simulink model "TxRxRFModel"  (R2018a)
settings: Solver=VariableStepAuto  StartTime=0.0  StopTime=10.0  RelTol=1e-3
InitFcn:
  | barker = comm.BarkerCode('SamplesPerFrame', 28, 'Length', 11);
  | seq = barker()+1;
  | M = 4;
  | hPSKModTrain   = comm.PSKModulator(M, ...
  |     'PhaseOffset',pi/4, ...
  |     'SymbolMapping','Binary');
  | xPreambleSeq = hPSKModTrain(seq);
  | 
  | 
  | %%%%%%%%%%%%
  | 
  | % AGC Preamble
  | reps = 5;
  | barker = comm.BarkerCode('SamplesPerFrame', 16, 'Length', 13);
  | seq = barker()+1;
  | %preamble = zeros(16*reps,1);
  | preambleFull = repmat(seq,reps,1);
  | rctFilt = comm.RaisedCosineTransmitFilter('FilterSpanInSymbols', 128,...
  | 'RolloffFactor',0.5,...
  | 'OutputSamplesPerSymbol',4);
  | preambleFullFilt = rctFilt(preambleFull);
  | 
  | %%%%%%%%%%%%
  | 
  | %RadioSampleRate = 1e6;
  | RadioSampleRate = 20e6;
  | RadioFrameLength = 1e5;
  | 
  | VibertiTracebackLength = 34+0;
  | numTrainingSamples = 250;
  | crc32Poly = [1 0 0 0 0 0 1 0 0 1 1 0 0 0 0 0 1 0 0 0 1 1 1 0 1 1 0 1 1 0 1 1 1];
  | crcDecodeLag = length(crc32Poly)-1+2;
  | 
  | %%%%%%%%%%%%
  | 
  | beta = 0.5;
  | span = 8;
  | sps = 4;
  | filterGain = 1;
  | coeff = rcosdesign(beta, span, sps, 'sqrt')*filterGain;
  | 
  | %%%%%%%%%%%%
  | 
  | samplesPerSymbol = 4;
  | maxPacketBits = 8*1500;
  | bItsPerSymbol = 2;
  | CodeRate = 2;
  | tailSymbols = 40;
  | maxPayloadSymbols = maxPacketBits*CodeRate/bItsPerSymbol+tailSymbols;
undefined symbols (not defined in the file or in its folder): ad9361_models, ad9361_preload, ad9361_rx, ad9361_tx, D, dBval, DCLeak_Matrix, designMultirateFIR, dfilt, doppler, errordlg, Frame, fuzz_val, GainImb_Matrix, IP2_Matrix, IP3_Matrix, magnitude
libraries: simulink x24, simrfV2elements x21, simrfV2util1 x9, dsparch4 x8, simrfV2junction1 x8, dspmlti4 x7, ad9361_private x3, simrfV2sources1 x3, dspmathops x3, commchan3 x2, hdlsllib x2, commdigbbndpm3 x2
(part 1 of 3)
settings Model: SimulationMode=accelerator  Creator=tcollins  LastModifiedBy=tcollins

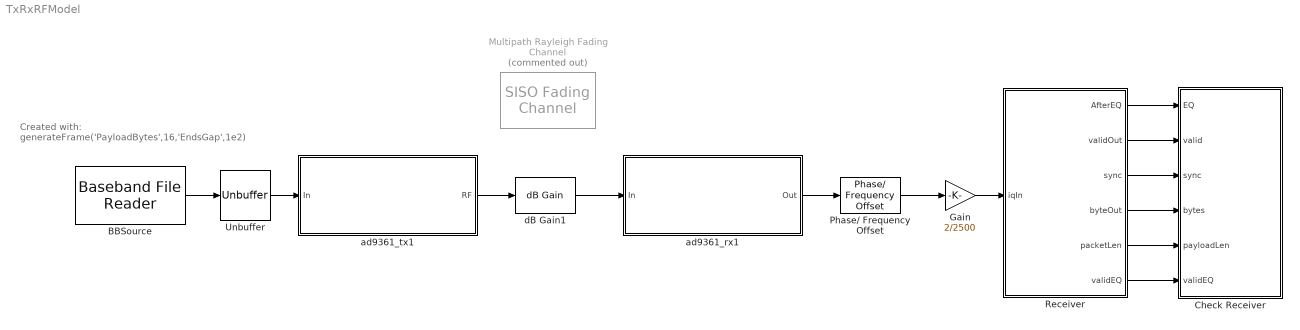
== system TxRxRFModel ==
  note: Created with:
      | generateFrame('PayloadBytes',16,'EndsGap',1e2)
  BBSource : commsource2/Baseband File Reader  Filename=refIQFrame.bb  InheritSampleTimeFromFile=off  SampleTime=100000/(RadioSampleRate)  SamplesPerFrame=100000  CyclicRepetition=on  FileEndOutputPort=off  SimulateUsing=Interpreted execution
      settings: SourceProductName=Communications Toolbox  SourceProductBaseCode=CM
  Check Receiver : Subsystem
  Gain : Gain  Gain=2/2500
  Multipath Rayleigh Fading Channel : commchan3/SISO Fading Channel  Commented=on  InheritSampleRate=on  SampleRate=1  PathDelays=[0 3e-8 5e-7]  AveragePathGains=[0 -20 -40]-60  NormalizePathGains=off  FadingDistribution=Rayleigh  KFactor=3  DirectPathDopplerShift=0  DirectPathInitialPhase=0  MaximumDopplerShift=5  DopplerSpectrum=doppler('Jakes')  ChannelInterpolationMethod=Polyphase  RandomStream=mt19937ar with seed  RandomNumGenerator=shr3cong  Seed=54873  PathGainsOutputPort=off  ChannelFilterDelayOutputPort=off  SimulateUsing=Code generation  Visualization=Off  PathsForDopplerDisplay=1  SamplesToDisplay=25%
      settings: SourceProductName=Communications Toolbox
  Phase/ Frequency Offset : commrflib2/Phase// Frequency Offset  phaseOffset=0  freqPort=off  freqOffset=1000
      settings: SourceProductName=Communications Toolbox
  Receiver : Subsystem  AncestorBlock=RxFloatingPointLibrary/Receiver
  Unbuffer : Unbuffer
  ad9361_rx1 : Subsystem  AncestorBlock=ad9361_models/ad9361_rx  LoadFcn=ad9361_preload(bdroot,'rx')  mask(ad9361_RX){TestSignal=Custom, LO=2e9, RF=2e9, Trf=1/160e6, RF_BW=160, IQ_rate=20}
      mask prompts: TestSignal "Filter Configuration:"; LO "LO Frequency [Hz]:"; RF "RF Center Frequency [Hz]:"; Trf "Step Size RF Simulation [s]:"; RF_BW "Input RF Bandwidth (MHz)"; IQ_rate "I/Q Sample Rate (MHz)"
      mask help: Model an Analog Devices ad9361 RF Receiver.
      mask init:
      | %load ad9361_rx_tables;
      | [ADIGainTable, ADIPhaseTable, ...
      |     DCLeak_Matrix, GainImb_Matrix, ...
      |     IP2_Matrix, IP3_Matrix] = ad9361_rx_gaintable(LO);
      | ad9361_rx_pars = ad9361_rx_initfcn(gcb,'Init');
      | ad9361_rx_pars = ad9361_rx_initfcn(gcb,'Build');
      mask Help:
      | Model an Analog Devices ad9361 RF Receiver. This model predicts thermal noise, spectral growth, LO carrier leakage and image signals, quantization noise in manual and slow attack control mode.
      | 
      | To change the automatic gain control mode, toggle the manual switch between manual mode and slow-attack control mode under the receiver mask. For manual mode, directly specify the index of the gain table in the constant block "manual index".
      | 
      | For signals with LTE 5MHz, LTE 10 MHz and LTE 20 MHz characteristics, the default configurations recommended by Analog Devices are directly available.
      | 
      | The filters are programmable. Use the Analog Devices Wizard App to custom design Filters. Select the option Custom in the Filter Configuration menu and click Design Filter button. The Filter Design app will open automatically. Make sure a receiver filter is designed instead of a transmitter filter. After designing the filter, click the button Export to Workspace in the App. The custom filter design is saved in the model set up. Next time a simulation is setup with custom filter configuration, the latest filter design is used.
      | 
      | Make sure that the input signal sample time and the expected step size of the RF simulation are the same. In case of a mismatch, an error is generated.
      mask TypeOptions TestSignal: 5MHz LTE | 10MHz LTE | 20MHz LTE | Custom
      mask Callback TestSignal:
      | % Set Mask visibilites and enables
      | ad9361_rx_mask_callbacks(gcb,'TestSignal')
      mask Callback Trf:
      | % block = gcb;
      | % p = Simulink.Mask.get(block);
      | % tmp = num2str(1/eval(get_param(gcb,'Trf'))/1e6,6);
      | % p.Parameters(5).Value = tmp;
      | set_param(gcb,'RF_BW',num2str(1/eval(get_param(gcb,'Trf'))/1e6,6));
      mask DialogControl ParameterGroupVar Prompt: ad9361 Receiver
      mask DialogControl Control2 Prompt: SpacerDesign
      mask DialogControl DesignFilter Prompt: Design Filter
      mask DialogControl DesignFilter Callback: ad9361_rx_initfcn(gcb,'DesignFilter');
      mask Display: text(0.5,0.5,'ad9361_RX','horizontalAlignment','center');
  ad9361_tx1 : Subsystem  AncestorBlock=ad9361_models/ad9361_tx  LoadFcn=ad9361_preload(bdroot,'tx')  mask(ad9361_TX){TestSignal=Custom, LOFreq=2e9, Att=0, IQ_rate=20, RF_BW=160}
      mask prompts: TestSignal "Filter Configuration:"; LOFreq "LO Frequency (Hz)"; Att "Attenuation (dB)"; IQ_rate "I/Q Sample Rate (MHz)"; RF_BW "RF Bandwidth (MHz)"
      mask help: Model an Analog Devices ad9361 RF Transmitter.
      mask init:
      | ad9361_tx_pars = ad9361_tx_initfcn(gcb,'Init');
      | ad9361_tx_pars = ad9361_tx_initfcn(gcb,'Build');
      mask Help:
      | Model an Analog Devices ad9361 RF Transmitter. This predicts thermal noise, phase noise, spectral growth, LO carrier leakage and image signals.
      | 
      | To change the attenuation value, modify the constant value in Attenuation block under the Transmitter mask. Transmitter attenuation is tunable between 0 to 80dB in steps of 0.25dB.
      | 
      | For signals with LTE 5MHz, LTE 10 MHz and LTE 20 MHz characteristics, the default configurations recommended by Analog Devices are directly available.
      | 
      | The filters are programmable. Use the Analog Devices Wizard App to custom design Filters. Select the option Custom in the Filter Configuration menu and click Design Filter button. The Filter Design App will open automatically. Make sure a transmitter filter is designed instead of a receiver filter. After designing the filter, click the button Export to Workspace in the App. The custom filter design is saved in the model set up. Next time a simulation is setup with custom filter configuration, the latest filter design is used.
      | 
      | Make sure that the input signal sample time and the expected signal sample time are the same. In case of a mismatch, an error is generated.
      mask TypeOptions TestSignal: 5MHz LTE | 10MHz LTE | 20MHz LTE | Custom
      mask Callback TestSignal:
      | % Control DesignFilter visibility
      | ad9361_tx_mask_callbacks(gcb,'TestSignal')
      mask DialogControl ParameterGroupVar Prompt: ad9361 Transmitter
      mask DialogControl DesignFilter Prompt: Design Filter
      mask DialogControl DesignFilter Callback: [~] = ad9361_tx_initfcn(gcb,'DesignFilter');
      mask DialogControl Control3 Prompt: SpacerDesign
      mask Display: text(0.5,0.5,'ad9361_TX','horizontalAlignment','center');
  dB Gain1 : dspmathops/dB Gain  dB=-60  intype=Amplitude
      settings: SourceProductName=DSP System Toolbox  SourceProductBaseCode=DS
  wires:
  BBSource/1 -> Unbuffer/1
  ad9361_tx1/1(RF) -> dB Gain1/1
  Unbuffer/1 -> ad9361_tx1/1(In)
  dB Gain1/1 -> ad9361_rx1/1(In)
  Phase/ Frequency Offset/1 -> Gain/1
  Receiver/1(AfterEQ) -> Check Receiver/1(EQ)
  Receiver/2(validOut) -> Check Receiver/2(valid)
  Receiver/3(sync) -> Check Receiver/3(sync)
  Receiver/4(byteOut) -> Check Receiver/4(bytes)
  Receiver/5(packetLen) -> Check Receiver/5(payloadLen)
  Receiver/6(validEQ) -> Check Receiver/6(validEQ)
  Gain/1 -> Receiver/1(iqIn)
  ad9361_rx1/1(Out) -> Phase/ Frequency Offset/1

== system TxRxRFModel/Check Receiver ==
  EQ : Inport
  valid : Inport  Port=2
  sync : Inport  Port=3
  bytes : Inport  Port=4
  payloadLen : Inport  Port=5
  validEQ : Inport  Port=6
  Constellation Diagram : Subsystem
  DMA Capture : MATLAB Function  TreatAsAtomicUnit=on
  wires:
  EQ/1 -> Constellation Diagram/1(In1)
  validEQ/1 -> Constellation Diagram/Enable
  bytes/1 -> DMA Capture/1(bytes)
  valid/1 -> DMA Capture/2(validOut)
  sync/1 -> DMA Capture/3(sync)
  payloadLen/1 -> DMA Capture/4(payloadLen)

== system TxRxRFModel/Receiver ==
  iqIn : Inport
  After SRRC : ConstellationDiagram
  CRC Check and DMA Pack : Subsystem
  Constellation Diagram : Subsystem
  Frame Recover : Subsystem
  From Radio : SpectrumAnalyzer
  Gardner Timing Recovery : Subsystem
  Raised Cosine Receive Filter : commfilt2/Raised Cosine Receive Filter  filtType=Square root  R=0.5  filtSpan=8  N=4  downFactor=1  downOffset=0  filterGain=1  RateOptions=Allow multirate processing  framing=Mute  checkCoeff=off  variableName=rcRxFilt  currentFiltSpan=8  D=(8)/2  inputOffset=0  sampMode=Mute  saveAsFlag=0  rateMode=Downsampling  checkGain=Normalized  launchFVT=on  roundingMode=Floor  overflowMode=off  coeffDataTypeStr=Inherit: Same word length as input  coeffMin=[]  coeffMax=[]  coeffLastDataTypeStr=Inherit: Same word length as input  accumDataTypeStr=Inherit: Same as product output  accumLastDataTypeStr=Inherit: Same as product output  outputDataTypeStr=Inherit: Same as accumulator  outputMin=[]  outputMax=[]  outputLastDataTypeStr=Inherit: Same as accumulator
  AfterEQ : Outport
  validOut : Outport  Port=2
  sync : Outport  Port=3
  byteOut : Outport  Port=4
  packetLen : Outport  Port=5
  validEQ : Outport  Port=6
  wires:
  Gardner Timing Recovery/1(dataOut) -> Constellation Diagram/1(In1), Frame Recover/1(dataIn)
  Gardner Timing Recovery/2(strobe) -> Constellation Diagram/Enable, Frame Recover/2(validIn), Frame Recover/Enable
  Raised Cosine Receive Filter/1 -> After SRRC/1, Gardner Timing Recovery/1(dataIn)
  iqIn/1 -> Raised Cosine Receive Filter/1
  Frame Recover/1(AfterEQ) -> AfterEQ/1
  Frame Recover/4(frameStart) -> CRC Check and DMA Pack/3(startData)
  Frame Recover/5(frameEnd) -> CRC Check and DMA Pack/4(endCRC)
  Frame Recover/3(data) -> CRC Check and DMA Pack/2(bits)
  Frame Recover/6(packetLen) -> CRC Check and DMA Pack/5(payloadLen)
  CRC Check and DMA Pack/2(validOut) -> validOut/1
  CRC Check and DMA Pack/1(byteOut) -> byteOut/1
  CRC Check and DMA Pack/3(sync) -> sync/1
  CRC Check and DMA Pack/4(payloadLenOut) -> packetLen/1
  Frame Recover/2(validOut) -> validEQ/1, CRC Check and DMA Pack/1(validIn)

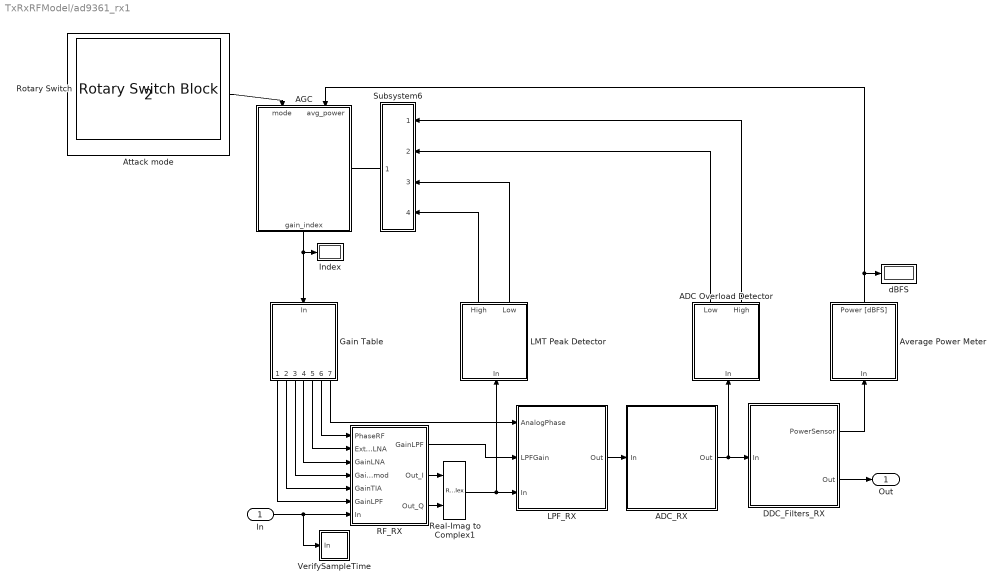
== system TxRxRFModel/ad9361_rx1 ==
  In : Inport
  ADC Overload Detector : Subsystem  mask{Ncycles=4, Lthreshold=47, Hthreshold=58}
      mask prompts: Ncycles "Number of Integration Cycles"; Lthreshold "Low Threshold"; Hthreshold "High Threshold"
      mask DialogControl DescGroupVar Prompt: ADC Overload Detector
  ADC_RX : Subsystem
  AGC : Stateflow chart  TreatAsAtomicUnit=on  mask{T=1, PeakOverLoadWait=1, SettlingDelay=32, FIR_Ts=ad9361_rx_pars.Tadc*ad9361_rx_pars.HB_interp, LMT_G_dec_fast=2, ADC_G_dec_fast=2, AGC_G_dec_fast=1, AGC_G_dec_slow=1, AGC_G_inc_fast=1, AGC_G_inc_slow=1, ManualGainIndex=76, C=3072 %approx 0.2ms, N_LMT_H=10, N_LMT_L=10, N_ADC_H=10, N_ADC_L=10, PT_HH=-8, PT_H=-10, PT_L=-12, PT_LL=-15, AGC_lock_level=-10, Max_Increase=5, EnableIncrGain=1, EnableGainIncAfterLock=1, AGC_attack_delay=10, EnergyDetectCount=32, IncrTime=5, LowPower=-13, PostLockStepSize=1, PowerMeasDuration=64, GainReset=Max Gain, GainOffset=5, EnergyLost=1, StrongerSignalThreshold=10, GainLockExitCount=8, Overrange=8}
      mask prompts: T "Extra delay margin [us]"; PeakOverLoadWait "Peak Overload Wait Time [cycles]"; SettlingDelay "Settling Delay Power Meter [cycles]"; FIR_Ts "FIR Input Clock Time"; LMT_G_dec_fast "LMT peak large decrement"; ADC_G_dec_fast "ADC peak large decrement"; AGC_G_dec_fast "Average Power large decrement"; AGC_G_dec_slow "Average Power small decrement"; AGC_G_inc_fast "Average Power large increment"; AGC_G_inc_slow "Average Power small increment"; ManualGainIndex "Gain Index"; C "Gain Update Counter [cycles]"; N_LMT_H "LMT Upper Count"; N_LMT_L "LMT Lower Count"; N_ADC_H "ADC Upper Count"; N_ADC_L "ADC Lower Count"; PT_HH "Outer Threshold High [dBFS]"; PT_H "Inner Threshold High [dBFS]"; PT_L "Inner Threshold Low [dBFS]"; PT_LL "Outer Threshold Low [dBFS]"; AGC_lock_level "AGC Lock Level [dBFS]"; Max_Increase "AGC Lock Level Max Increase [Index]"; EnableIncrGain "Enable Gain Increment [0/1]"; EnableGainIncAfterLock "Enable Gain Increment After Gain Lock [0/1]"; AGC_attack_delay "Attack delay [us]"; EnergyDetectCount "Energy Detect Count [cycles]"; IncrTime "Increment Time [cycles]"; LowPower "Low Power Threshold"; PostLockStepSize "Post Lock Level Step Size [Index]"; PowerMeasDuration "Power Measurement Duration - State 5 [cycles]"; GainReset "Gain Index When Reset"; GainOffset "Optimize Gain Offset"; EnergyLost "Energy Lost Level [dB]"; StrongerSignalThreshold "Stronger Signal Threshold [dB]"; GainLockExitCount "Gain Lock Exit Count [cycles]"; Overrange "Overrange Count [Events]"
      mask init:
      | EnergyDetectCount = EnergyDetectCount*FIR_Ts;
      | C = C*FIR_Ts;
      | SettlingDelay = SettlingDelay*FIR_Ts;
      | PeakOverLoadWait = PeakOverLoadWait*FIR_Ts;
      | PowerMeasDuration = PowerMeasDuration*FIR_Ts;
      | IncrTime = IncrTime*FIR_Ts;
      | 
      | tmp = get_param(gcb,'parent');
      | n = get_param([tmp, '/Average Power Meter'], 'Ncycles');
      | DecPowerMeasDuration = str2num(n)*FIR_Ts;
  Attack mode : Constant  Value=2  SampleTime=-1
      mask Display: disp(' ')
  Average Power Meter : Subsystem  mask{Ncycles=64}
      mask prompts: Ncycles "Number of Integration Cycles"
      mask DialogControl DescGroupVar Prompt: Average Power Meter
  DDC_Filters_RX : Subsystem
  Gain Table : Subsystem
  "Index " : Display
  LMT Peak Detector : Subsystem  mask{HThreshold=800, LThreshold=704}
      mask prompts: HThreshold "High Threshold [mV]"; LThreshold "Low Threshold [mV]"
      mask DialogControl DescGroupVar Prompt: LMT Peak Detector
  LPF_RX : Subsystem
  RF_RX : Subsystem  mask{RF=RF, LO=LO, Tstep=Trf}
      mask prompts: RF "Center Frequency [Hz]"; LO "LO Frequency [Hz]"; Tstep "Sample Time [s]"
      mask init:
      | freq = [0.8e9, 2.4e9, 5.5e9];
      | nf   = [2,     3,     3.8];
      | NF   = interp1(freq, nf, LO,'linear','extrap');
      | 
      | if length(unique([RF LO])) == 2
      |     HB = [3 1];
      | else
      |     HB = 3;
      | end
      mask DialogControl DescGroupVar Prompt: ad9361 Receiver RF Front End
  Real-Imag to Complex1 : RealImagToComplex
  Rotary Switch : RotarySwitchBlock  WebBlockId=5998  LabelPosition=Hide
      settings: Values={{'Slow', 'Manual', 'Fast'}, [0 1 2]}
  Subsystem6 : Subsystem  mask{NCyclesADC=4}
      mask prompts: NCyclesADC "ADC Integration Cycles"
  VerifySampleTime : Subsystem
  dBFS : Display
  Out : Outport
  wires:
  Gain Table/6(RF phase) -> RF_RX/1(PhaseRF)
  RF_RX/2(Out_I) -> Real-Imag to Complex1/1
  RF_RX/3(Out_Q) -> Real-Imag to Complex1/2
  Real-Imag to Complex1/1 -> LMT Peak Detector/1(In), LPF_RX/3(In)
  Gain Table/2(tia) -> RF_RX/5(GainTIA)
  Gain Table/3(demod) -> RF_RX/4(GainDemod)
  Gain Table/4(lna) -> RF_RX/3(GainLNA)
  LPF_RX/1(Out) -> ADC_RX/1(In)
  LMT Peak Detector/2(Low) -> Subsystem6/3(LMT_L)
  Gain Table/1(lpf) -> RF_RX/6(GainLPF)
  DDC_Filters_RX/1(PowerSensor) -> Average Power Meter/1(In)
  ADC Overload Detector/2(High) -> Subsystem6/1(ADC_H)
  LMT Peak Detector/1(High) -> Subsystem6/4(LMT_H)
  ADC Overload Detector/1(Low) -> Subsystem6/2(ADC_L)
  DDC_Filters_RX/2(Out) -> Out/1
  In/1 -> RF_RX/7(In), VerifySampleTime/1(In)
  Subsystem6/1(Peak) -> AGC/Trigger
  RF_RX/1("GainLPF ") -> LPF_RX/2(LPFGain)
  Gain Table/5(External LNA) -> RF_RX/2(ExternalLNA)
  Attack mode/1 -> AGC/1(mode)
  Average Power Meter/1(Power [dBFS]) -> dBFS/1, AGC/2(avg_power)
  AGC/1(gain_index) -> "Index "/1, Gain Table/1(In)
  ADC_RX/1(Out) -> DDC_Filters_RX/1(In), ADC Overload Detector/1(In)
  Gain Table/7(Analog phase) -> LPF_RX/1(AnalogPhase)

== system TxRxRFModel/ad9361_tx1 ==
  In : Inport
  Analog_Filters_TX : Subsystem
  Attenuation : Constant  Value=Att
  DUC_Filters_TX : Subsystem
  RF_TX : Subsystem  mask{RF=LOFreq, Tstep=ad9361_tx_pars.Tduc}
      mask prompts: RF "Center Frequency (Hz)"; Tstep "Sample Time (s)"
      mask init:
      | Gain = interp1([800e6, 2.4e9, 5.5e9], [0, 0, -1]+8.3, RF, 'linear', 'extrap');
      | 
      | % Output referred IP3
      | oip3_800MHz = [23, 25, 10, 10];
      | oip3_2p4GHz = [19, 18,  6,  6];
      | oip3_5p5GHz = [17, 13,  2,  2];
      | Att_ip3     = [0 4 20 80];
      | if RF < 1.6e9
      |     OIP3v = oip3_800MHz;
      | elseif RF < 4e9
      |     OIP3v = oip3_2p4GHz;
      | else
      |     OIP3v = oip3_5p5GHz;
      | end
      | % Attenuation measurement data (dB)
      | Attdata  = [0  10  20  30  40  50   60   70   80];
      | % LO carrier leakage (dBm)
      | LO_leak  = ([-58 -52 -60 -71 -81 -82 -101 -102 -100]-Gain-6)/10;
      | % Gain imbalance (dBc)
      | Gain_imb = [-55.5 -66.2 -53.5 -57.5 -44.5 -46.3 -54.2 -46.1 -34.3]/20;
      | % Phase noise characteristics (dBm/Hz)
      | freqPN   = [1e3, 1e4, 1e5, 1e6, 3e6];
      | PN       = [-95, -110, -110, -125, -157]; 
      | % Thermal noise floor (dBm/Hz)
      | NF       = interp1([800e6, 2.4e9, 5.5e9], [17, 18, 22.5], RF, 'linear', 'extrap');
      | 
      | set_param([gcb '/Configuration'], 'AddNoise','on');
      mask DialogControl Container1 Prompt: ad9361 Transmitter RF Front End
  VerifySampleTime : Subsystem
  RF : Outport
  wires:
  Analog_Filters_TX/1(Real) -> RF_TX/1(In_I)
  Analog_Filters_TX/2(Imaginary) -> RF_TX/2(In_Q)
  In/1 -> VerifySampleTime/1(In), DUC_Filters_TX/1(In)
  Attenuation/1 -> RF_TX/3(Attenuation)
  DUC_Filters_TX/1(Out) -> Analog_Filters_TX/1(In)
  RF_TX/1(Out) -> RF/1

== system TxRxRFModel/Check Receiver/Constellation Diagram ==
  In1 : Inport
  Enable : EnablePort
  After EQ (Outside) : ConstellationDiagram
  wires:
  In1/1 -> After EQ (Outside)/1

== system TxRxRFModel/Receiver/CRC Check and DMA Pack ==
  validIn : Inport
  bits : Inport  Port=2
  startData : Inport  Port=3
  endCRC : Inport  Port=4
  payloadLen : Inport  Port=5
  CRC Check ES : Subsystem
  CRC Decode Lag : Delay  DelayLength=crcDecodeLag+2
  DMA Interface : Subsystem
  Delay : Delay  DelayLength=1
  Logical Operator : Logic  AllPortsSameDT=off  OutDataTypeStr=boolean
  overdrive : MATLAB Function  TreatAsAtomicUnit=on
  byteOut : Outport
  validOut : Outport  Port=2
  sync : Outport  Port=3
  payloadLenOut : Outport  Port=4
  wires:
  DMA Interface/2(validOut) -> validOut/1
  DMA Interface/1(byteOut) -> byteOut/1
  bits/1 -> CRC Check ES/2(Bits)
  DMA Interface/3(sync) -> sync/1
  payloadLen/1 -> CRC Check ES/5(payloadLen)
  startData/1 -> CRC Check ES/4(StartData)
  endCRC/1 -> CRC Check ES/3(endCRC)
  CRC Check ES/1(dataOut) -> DMA Interface/1(bitIn)
  CRC Check ES/2(startOut) -> DMA Interface/2(startIn)
  CRC Check ES/3(endOut) -> DMA Interface/3(endIn), Delay/1
  Logical Operator/1 -> DMA Interface/4(validIn)
  CRC Check ES/5(err) -> DMA Interface/5(err)
  CRC Check ES/6(payloadLenOut) -> DMA Interface/6(payloadLen)
  CRC Decode Lag/1 -> Logical Operator/1
  CRC Check ES/4(validOut) -> Logical Operator/2
  validIn/1 -> CRC Check ES/1(Valid), CRC Decode Lag/1, overdrive/1(validIn)
  Delay/1 -> overdrive/2(endIn)
  DMA Interface/4(payloadLenOut) -> payloadLenOut/1
  overdrive/1(enableCRC) -> CRC Check ES/Enable

== system TxRxRFModel/Receiver/Constellation Diagram ==
  In1 : Inport
  Enable : EnablePort
  After Timing Recovery : ConstellationDiagram
  wires:
  In1/1 -> After Timing Recovery/1

== system TxRxRFModel/Receiver/Frame Recover ==
  dataIn : Inport
  validIn : Inport  Port=2
  Enable : EnablePort
  After Frequency Recovery : ConstellationDiagram
  Barker Locate : Subsystem  mask{Threshold=0.8}
  Enable Equalizer and Packet Decode (Latch) : MATLAB Function  TreatAsAtomicUnit=on
  Equalization and Demodulation : Subsystem
  Frequency Recovery : Subsystem
  AfterEQ : Outport
  validOut : Outport  Port=2  OutputWhenDisabled=reset  InitialOutput=0
  data : Outport  Port=3
  frameStart : Outport  Port=4
  frameEnd : Outport  Port=5
  packetLen : Outport  Port=6
  wires:
  validIn/1 -> Frequency Recovery/2(validIn)
  dataIn/1 -> Frequency Recovery/1(dataIn)
  Frequency Recovery/2(validOut) -> Barker Locate/2(enableIn)
  Frequency Recovery/1(dataOut) -> After Frequency Recovery/1, Barker Locate/1(In1)
  Equalization and Demodulation/5(packLen) -> packetLen/1
  Barker Locate/1(Detector) -> Enable Equalizer and Packet Decode (Latch)/1(start), Equalization and Demodulation/1(Trigger)
  Barker Locate/3(enableOut) -> Enable Equalizer and Packet Decode (Latch)/2(validIn)
  Barker Locate/2(Signal) -> Equalization and Demodulation/2(Data)
  Enable Equalizer and Packet Decode (Latch)/1(enable) -> Equalization and Demodulation/Enable
  Equalization and Demodulation/3(crcEnd) -> frameEnd/1
  Equalization and Demodulation/2(validOut) -> validOut/1
  Equalization and Demodulation/1(AfterEQ) -> AfterEQ/1
  Equalization and Demodulation/4(dataOut) -> data/1
  Equalization and Demodulation/6(frameStart) -> frameStart/1

== system TxRxRFModel/Receiver/Gardner Timing Recovery ==
  dataIn : Inport
  Delay : Delay  DelayLength=1
  Delay1 : Delay  DelayLength=1
  Gardner TED Blocks : Subsystem
  InterpControl_Blocks1 : Subsystem
  Interpolator : Subsystem
  LoopFilter : Subsystem  mask{zeta=sqrt(2), BnTs=0.01, Kp=2.7}
      mask prompts: zeta "DampingFactor"; BnTs "NormalizedLoopBandwidth"; Kp "DetectionGain"
      mask init:
      | K0 = -1;
      | SPS = 4;
      | theta = BnTs/SPS/(zeta + 0.25/zeta);
      | d  = (1 + 2*zeta*theta + theta^2) * K0 * Kp;
      | ProportionalGain = (4*zeta*theta) /d;
      | IntegratorGain   = (4*theta*theta)/d;
  dataOut : Outport  InitialOutput=0
  strobe : Outport  Port=2  InitialOutput=false
  wires:
  Delay1/1 -> Gardner TED Blocks/2(strobe), strobe/1
  Delay/1 -> Interpolator/2(mu)
  Interpolator/1(Out1) -> Gardner TED Blocks/1(data), dataOut/1
  Gardner TED Blocks/1(e) -> LoopFilter/1(e)
  InterpControl_Blocks1/1(strobe) -> Delay1/1
  InterpControl_Blocks1/2(mu) -> Delay/1
  LoopFilter/1(v) -> InterpControl_Blocks1/1(e)
  dataIn/1 -> Interpolator/1(In1)

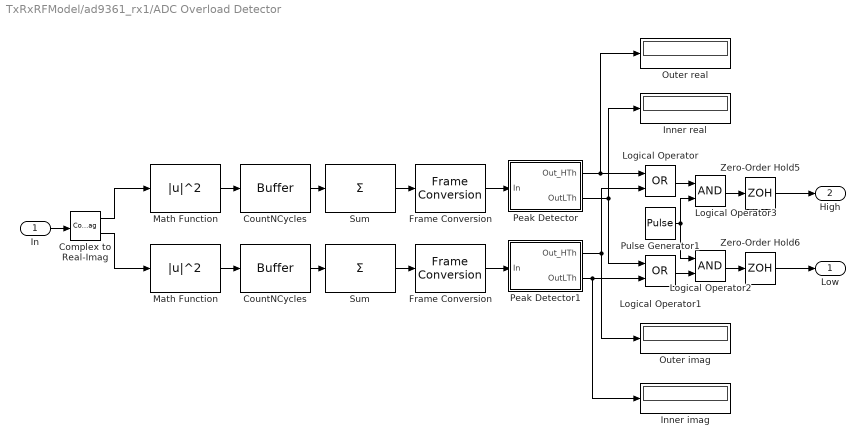
== system TxRxRFModel/ad9361_rx1/ADC Overload Detector ==
  In : Inport
  Complex to Real-Imag : ComplexToRealImag
  CountNCycles : Buffer  N=Ncycles
  "CountNCycles " : Buffer  N=Ncycles
  Frame Conversion : FrameConversion  OutFrame=Sample-based
  "Frame Conversion " : FrameConversion  OutFrame=Sample-based
  Inner imag : Display
  Inner real : Display
  Logical Operator : Logic  Operator=OR  AllPortsSameDT=off  OutDataTypeStr=boolean
  Logical Operator1 : Logic  Operator=OR  AllPortsSameDT=off  OutDataTypeStr=boolean
  Logical Operator2 : Logic  AllPortsSameDT=off  OutDataTypeStr=boolean
  Logical Operator3 : Logic  AllPortsSameDT=off  OutDataTypeStr=boolean
  Math Function : Math  Operator=magnitude^2  SaturateOnIntegerOverflow=on
  "Math Function " : Math  Operator=magnitude^2  SaturateOnIntegerOverflow=on
  Outer imag : Display
  Outer real : Display
  Peak Detector : Subsystem  mask{HThreshold=Hthreshold, LThreshold=Lthreshold}
      mask prompts: HThreshold "High Threshold (bit string) <4:0>"; LThreshold "Low Threshold (bit string) <4:0>"
  Peak Detector1 : Subsystem  mask{HThreshold=Hthreshold, LThreshold=Lthreshold}
      mask prompts: HThreshold "High Threshold (bit string) <4:0>"; LThreshold "Low Threshold (bit string) <4:0>"
  Pulse Generator1 : DiscretePulseGenerator  SampleTime=ad9361_rx_pars.Tadc*Ncycles
  Sum : Sum  Inputs=+
  "Sum " : Sum  Inputs=+
  Zero-Order Hold5 : ZeroOrderHold  SampleTime=Trf
  Zero-Order Hold6 : ZeroOrderHold  SampleTime=Trf
  Low : Outport
  High : Outport  Port=2
  wires:
  Math Function/1 -> CountNCycles/1
  CountNCycles/1 -> Sum/1
  Sum/1 -> Frame Conversion/1
  Frame Conversion/1 -> Peak Detector/1(In)
  In/1 -> Complex to Real-Imag/1
  "Math Function "/1 -> "CountNCycles "/1
  "CountNCycles "/1 -> "Sum "/1
  "Sum "/1 -> "Frame Conversion "/1
  "Frame Conversion "/1 -> Peak Detector1/1(In)
  Peak Detector/2(OutLTh) -> Logical Operator1/1, Inner real/1
  Peak Detector/1(Out_HTh) -> Outer real/1, Logical Operator/1
  Peak Detector1/1(Out_HTh) -> Logical Operator/2, Outer imag/1
  Peak Detector1/2(OutLTh) -> Inner imag/1, Logical Operator1/2
  Complex to Real-Imag/1 -> Math Function/1
  Complex to Real-Imag/2 -> "Math Function "/1
  Logical Operator/1 -> Logical Operator3/1
  Logical Operator2/1 -> Zero-Order Hold6/1
  Logical Operator1/1 -> Logical Operator2/2
  Logical Operator3/1 -> Zero-Order Hold5/1
  Pulse Generator1/1 -> Logical Operator2/1, Logical Operator3/2
  Zero-Order Hold5/1 -> High/1
  Zero-Order Hold6/1 -> Low/1

== system TxRxRFModel/ad9361_rx1/ADC_RX ==
  In : Inport
  ADC_I : Subsystem
  ADC_Q : Subsystem
  Complex to Real-Imag1 : ComplexToRealImag
  Real-Imag to Complex : RealImagToComplex
  Out : Outport
  wires:
  Complex to Real-Imag1/1 -> ADC_I/1(In)
  Complex to Real-Imag1/2 -> ADC_Q/1(In)
  In/1 -> Complex to Real-Imag1/1
  Real-Imag to Complex/1 -> Out/1
  ADC_I/1(Out) -> Real-Imag to Complex/1
  ADC_Q/1(Out) -> Real-Imag to Complex/2

== system TxRxRFModel/ad9361_rx1/Average Power Meter ==
  In : Inport
  Max saturation power dBm : Constant  Value=20*log10(4)+30
  Quantizer : Quantizer
  RMS : Subsystem
  Saturation : Saturate  UpperLimit=0  LowerLimit=-63.5
  Subtract : Sum  Inputs=+-
  dB Conversion : Subsystem  mask(dB Conversion){dBtype=dBm, intype=Amplitude, R=1, fuzz=on}
      mask prompts: dBtype "Convert to:"; intype "Input signal:"; R "Load resistance (ohms):"; fuzz "Add eps to input to protect against  "log(0) = -inf""
      mask help: Convert input of watts or volts to decibels. Voltage inputs are first converted to power relative to the specified load resistance, where P = (V^2)/R. When converting to dB, the reference power is 1 W. When converting to dBm, the reference power is 1 mW.
      mask init:
      | [str fuzz_val dBval] = dspblkdb2('init');
      | dspblkdb2('checkparam');
      | dspblkdb2('update');
      mask Help: eval('blocksethelp');
      mask TypeOptions dBtype: dB | dBm
      mask Callback dBtype: dspblkdb2
      mask TypeOptions intype: Power | Amplitude
      mask Callback intype: dspblkdb2
      mask Display: disp(str)
  Power [dBFS] : Outport
  wires:
  Max saturation power dBm/1 -> Subtract/2
  Subtract/1 -> Quantizer/1
  Quantizer/1 -> Saturation/1
  dB Conversion/1(out) -> Subtract/1
  In/1 -> RMS/1(In)
  RMS/1(Out) -> dB Conversion/1(in)
  Saturation/1 -> Power [dBFS]/1

== system TxRxRFModel/ad9361_rx1/DDC_Filters_RX ==
  In : Inport
  Data Type Conversion1 : DataTypeConversion  OutDataTypeStr=double
  Data Type Conversion2 : DataTypeConversion  OutDataTypeStr=double
  FIR Decimation : dspmlti4/FIR Decimation  FilterSource=Filter object  h=fir1(35,0.4)  D=2  filtStruct=Direct form  FilterObject=ad9361_rx_pars.Hmd_rx  framing=Allow multirate processing  inputOffset=0  outputBufInitCond=0  roundingMode=Floor  overflowMode=off  firstCoeffDataTypeStr=Inherit: Same word length as input  firstCoeffMin=[]  firstCoeffMax=[]  firstCoeffLastDataTypeStr=Inherit: Same word length as input  outputDataTypeStr=Inherit: Same as accumulator  outputMin=[]  outputMax=[]  outputLastDataTypeStr=Inherit: Same as accumulator
  Gain : Gain  Gain=1/4
  Gain1 : Gain  Gain=4
  Hm1 : dspmlti4/FIR Decimation  FilterSource=Filter object  h=designMultirateFIR(1,2)  D=2  filtStruct=Direct form  FilterObject=ad9361_rx_pars.Hm1_rx  framing=Enforce single-rate processing  inputOffset=0  outputBufInitCond=0  roundingMode=Floor  overflowMode=off  firstCoeffDataTypeStr=Inherit: Same word length as input  firstCoeffMin=[]  firstCoeffMax=[]  firstCoeffLastDataTypeStr=Inherit: Same word length as input  outputDataTypeStr=Inherit: Same as accumulator  outputMin=[]  outputMax=[]  outputLastDataTypeStr=Inherit: Same as accumulator
  Hm2 : ad9361_private/ConvertAndFIR  DataTypeOut=fixdt(1,16,14)  FilterObj=ad9361_rx_pars.Hm2_rx
  Hm3 : dspmlti4/FIR Decimation  FilterSource=Filter object  h=designMultirateFIR(1,2)  D=2  filtStruct=Direct form  FilterObject=ad9361_rx_pars.Hm3_rx  framing=Enforce single-rate processing  inputOffset=0  outputBufInitCond=0  roundingMode=Floor  overflowMode=off  firstCoeffDataTypeStr=Inherit: Same word length as input  firstCoeffMin=[]  firstCoeffMax=[]  firstCoeffLastDataTypeStr=Inherit: Same word length as input  outputDataTypeStr=Inherit: Same as accumulator  outputMin=[]  outputMax=[]  outputLastDataTypeStr=Inherit: Same as accumulator
  Hm4 : ad9361_private/Short  SystemSampleTime=-1  VariantControl=ad9361_tx_hm1Filt==0
  dBFS : Subsystem
  PowerSensor : Outport
  Out : Outport  Port=2
  wires:
  In/1 -> Gain/1
  Hm4/1 -> Hm3/1
  Hm3/1 -> Hm2/1
  Hm2/1 -> Hm1/1
  FIR Decimation/1 -> Data Type Conversion2/1
  Gain/1 -> Hm4/1
  Data Type Conversion1/1 -> Gain1/1
  Gain1/1 -> PowerSensor/1
  Hm1/1 -> FIR Decimation/1, Data Type Conversion1/1
  Data Type Conversion2/1 -> dBFS/1(In)
  dBFS/1(Out) -> Out/1

== system TxRxRFModel/ad9361_rx1/Gain Table ==
  In : Inport
  Add : Sum
  Add1 : Sum
  Delay1 : Delay  DelayLength=1  InitialCondition=76  SampleTime=Trf
  Demux : Demux  Outputs=6
  Demux1 : Demux  Outputs=5
  Direct Lookup Gain Table (n-D) : LookupNDDirect  InputsSelectThisObjectFromTable=Vector  Table=ADIGainTable'
  Direct Lookup Phase Table (n-D)1 : LookupNDDirect  InputsSelectThisObjectFromTable=Vector  Table=ADIPhaseTable'
  Index : Terminator
  Index1 : Terminator
  lpf : Outport
  tia : Outport  Port=2
  demod : Outport  Port=3
  lna : Outport  Port=4
  External LNA : Outport  Port=5
  RF phase : Outport  Port=6
  Analog phase : Outport  Port=7
  wires:
  Demux/3 -> demod/1
  Demux/2 -> lna/1
  Demux/4 -> tia/1
  Demux/5 -> lpf/1
  In/1 -> Delay1/1
  Delay1/1 -> Direct Lookup Phase Table (n-D)1/1, Direct Lookup Gain Table (n-D)/1
  Direct Lookup Gain Table (n-D)/1 -> Demux/1
  Demux/6 -> External LNA/1
  Demux/1 -> Index/1
  Direct Lookup Phase Table (n-D)1/1 -> Demux1/1
  Demux1/1 -> Index1/1
  Demux1/2 -> Add/1
  Demux1/3 -> Add/2
  Demux1/4 -> Add1/1
  Demux1/5 -> Add1/2
  Add/1 -> RF phase/1
  Add1/1 -> Analog phase/1

== system TxRxRFModel/ad9361_rx1/LMT Peak Detector ==
  In : Inport
  Abs : Abs
  HTh : Constant  Value=HThreshold*1e-3
  "High " : Display
  HighThreshold : RelationalOperator  OutDataTypeStr=boolean  RndMeth=Nearest
  LTh : Constant  Value=LThreshold*1e-3
  Logical Operator : Logic  AllPortsSameDT=off  OutDataTypeStr=boolean
  Logical Operator1 : Logic  AllPortsSameDT=off  OutDataTypeStr=boolean
  "Low " : Display
  LowThreshold : RelationalOperator  OutDataTypeStr=boolean  RndMeth=Nearest
  Pulse Generator2 : DiscretePulseGenerator  SampleTime=Trf
  High : Outport  SampleTime=Trf
  Low : Outport  Port=2  SampleTime=Trf
  wires:
  LTh/1 -> LowThreshold/2
  Abs/1 -> HighThreshold/1, LowThreshold/1
  HTh/1 -> HighThreshold/2
  In/1 -> Abs/1
  HighThreshold/1 -> Logical Operator1/1, "High "/1
  LowThreshold/1 -> Logical Operator/2, "Low "/1
  Pulse Generator2/1 -> Logical Operator1/2, Logical Operator/1
  Logical Operator1/1 -> High/1
  Logical Operator/1 -> Low/1

== system TxRxRFModel/ad9361_rx1/LPF_RX ==
  AnalogPhase : Inport
  LPFGain : Inport  Port=2
  In : Inport  Port=3
  Complex Phase Shift : commutil2/Complex Phase Shift
      settings: SourceProductName=Communications Toolbox  SourceProductBaseCode=CM
  Complex to Real-Imag : ComplexToRealImag
  Gain : Product
  LPF_I : dsparch4/Analog Filter Design  method=Butterworth  filttype=Lowpass  N=3  Wlo=1.4*ad9361_rx_pars.Fpass*2*pi  Whi=80  Rp=2  Rs=40
  "LPF_Q " : dsparch4/Analog Filter Design  method=Butterworth  filttype=Lowpass  N=3  Wlo=1.4*ad9361_rx_pars.Fpass*2*pi  Whi=80  Rp=2  Rs=40
  Phase[deg] : Display
  Real-Imag to Complex1 : RealImagToComplex
  ToRadians : Gain  Gain=pi/180
  dB2lin : Subsystem
  Out : Outport
  wires:
  Complex to Real-Imag/1 -> LPF_I/1
  Real-Imag to Complex1/1 -> Out/1
  Complex Phase Shift/1 -> Gain/2
  LPFGain/1 -> dB2lin/1(In)
  Gain/1 -> Complex to Real-Imag/1
  dB2lin/1(Out) -> Gain/1
  "LPF_Q "/1 -> Real-Imag to Complex1/2
  LPF_I/1 -> Real-Imag to Complex1/1
  Complex to Real-Imag/2 -> "LPF_Q "/1
  In/1 -> Complex Phase Shift/1
  AnalogPhase/1 -> Phase[deg]/1, ToRadians/1
  ToRadians/1 -> Complex Phase Shift/2

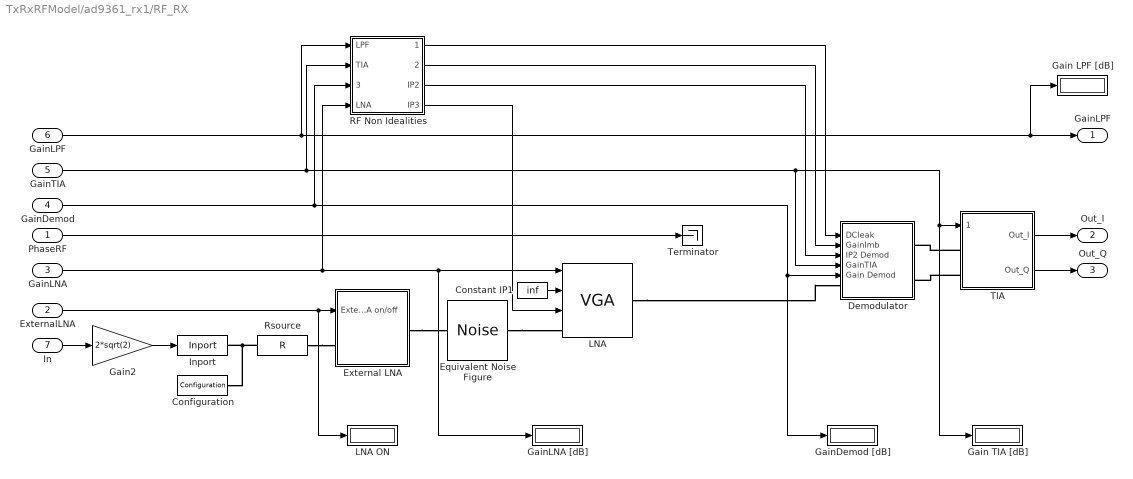
== system TxRxRFModel/ad9361_rx1/RF_RX ==
  PhaseRF : Inport
  ExternalLNA : Inport  Port=2
  GainLNA : Inport  Port=3
  GainDemod : Inport  Port=4
  GainTIA : Inport  Port=5
  GainLPF : Inport  Port=6
  In : Inport  Port=7
  Configuration : simrfV2util1/Configuration  AutoFreq=off  Tones=unique([RF LO]) Hz  Harmonics=HB  NormalizeCarrierPower=on  SolverType=Auto  UseCCode=on  StepSize=Tstep s  AddNoise=on  defaultRNG=on  Seed=0  Temperature=290.0 K  SolverDelFlag=0  AbsTol=1e-6  RelTol=1e-3  MaxIter=10  ErrorEstimationType=2-norm over all variables
      settings: SourceProductName=RF Blockset  SourceProductBaseCode=RB
  Constant IP1 : Constant  Value=inf
  Demodulator : Subsystem
  Equivalent Noise Figure : simrfV2sources1/Noise  SimulinkInputSignalType=Ideal voltage  NoiseType=White  NoisePSD=4*1.381e-23*290*50*10^(NF/10)  CarrierFreq=fc_RF Hz  AutoImpulseLength=on  ImpulseLength=1e-10 s  InternalGrounding=off
      settings: SourceProductName=RF Blockset  SourceProductBaseCode=RB
  External LNA : Subsystem
  Gain LPF [dB] : Display
  Gain TIA [dB] : Display
  Gain2 : Gain  Gain=2*sqrt(2)
  GainDemod [dB] : Display
  GainLNA [dB] : Display
  Inport : simrfV2util1/Inport  SimulinkInputSignalType=Ideal voltage  CarrierFreq=RF Hz  ZS=0  InternalGrounding=on
      settings: SourceProductName=RF Blockset  SourceProductBaseCode=RB
  LNA : simrfV2elements/VGA  classname=vga  Zin=50  Zout=50  IO=Input  InternalGrounding=on
      settings: SourceProductName=RF Blockset  SourceProductBaseCode=RB
  LNA ON : Display
  RF Non Idealities : Subsystem
  Rsource : simrfV2elements/R  classname=resistor  Resistance=50 Ohm  AddNoise=on
      settings: SourceProductName=RF Blockset  SourceProductBaseCode=RB
  TIA : Subsystem
  Terminator : Terminator
  "GainLPF " : Outport
  Out_I : Outport  Port=2
  Out_Q : Outport  Port=3
  wires:
  PhaseRF/1 -> Terminator/1
  In/1 -> Gain2/1
  Gain2/1 -> Inport/1
  TIA/1(Out_I) -> Out_I/1
  GainLPF/1 -> "GainLPF "/1, Gain LPF [dB]/1, RF Non Idealities/1(LPF)
  GainTIA/1 -> Demodulator/4(GainTIA), Gain TIA [dB]/1, TIA/1(Gain TIA), RF Non Idealities/2(TIA)
  GainDemod/1 -> Demodulator/5(Gain Demod), GainDemod [dB]/1, RF Non Idealities/3(Demod)
  GainLNA/1 -> RF Non Idealities/4(LNA), LNA/1, GainLNA [dB]/1
  RF Non Idealities/1(DCLeakage) -> Demodulator/1(DCleak)
  RF Non Idealities/3(IP2) -> Demodulator/3(IP2 Demod)
  RF Non Idealities/4(IP3) -> LNA/3
  Constant IP1/1 -> LNA/2
  ExternalLNA/1 -> LNA ON/1, External LNA/1(ExternalLNA on/off)
  RF Non Idealities/2(GainImbalance) -> Demodulator/2(GainImb)
  TIA/2(Out_Q) -> Out_Q/1
  connections:
  LNA/RConn1 -- Demodulator/LConn1
  Rsource/RConn1 -- Configuration/LConn1 -- Inport/RConn1
  Equivalent Noise Figure/LConn1 -- LNA/LConn1
  TIA/LConn2 -- Demodulator/RConn2
  TIA/LConn1 -- Demodulator/RConn1
  Rsource/LConn1 -- External LNA/LConn1
  External LNA/RConn1 -- Equivalent Noise Figure/RConn1

== system TxRxRFModel/ad9361_rx1/Subsystem6 ==
  ADC_H : Inport
  ADC_L : Inport  Port=2
  LMT_L : Inport  Port=3
  LMT_H : Inport  Port=4
  Data Type Conversion : DataTypeConversion  OutDataTypeStr=boolean
  Logical Operator : Logic  Operator=OR  AllPortsSameDT=off  OutDataTypeStr=boolean
  Mux : Mux  Inputs=5
  Subsystem1 : Subsystem
  Wblk5 : Subsystem
  Wblk6 : Subsystem
  Wblk7 : Subsystem
  Peak : Outport
  wires:
  LMT_L/1 -> Wblk7/1(Win)
  Logical Operator/1 -> Wblk7/2(Sin), Wblk6/2(Sin)
  Wblk7/1(Wout) -> Mux/3  "LMT_L"
  Wblk6/1(Wout) -> Mux/2  "ADC_L"
  Wblk5/1(Wout) -> Mux/1, Logical Operator/1  "ADC_H"
  Subsystem1/1(START) -> Data Type Conversion/1
  Data Type Conversion/1 -> Mux/5  "Event"
  ADC_L/1 -> Wblk6/1(Win)
  ADC_H/1 -> Wblk5/1(Win)
  LMT_H/1 -> Wblk5/2(Sin), Mux/4, Logical Operator/2  "LMT_H"
  Mux/1 -> Peak/1

== system TxRxRFModel/ad9361_rx1/VerifySampleTime ==
  In : Inport
  Abs : Abs
  Assertion : Assertion  AssertionFailFcn=errordlg('Test signal sample time and RF simulation step size are not consistent');
  Compare To Constant : simulink/Logic and Bit Operations/Compare To Constant  relop=<=  const=eps(1/Trf)  OutDataTypeStr=boolean
  Constant : Constant  Value=Trf
  Subtract : Sum  Inputs=+-
  Weighted Sample Time : SampleTimeMath  TsampMathOp=Ts Only
  wires:
  Compare To Constant/1 -> Assertion/1
  Abs/1 -> Compare To Constant/1
  Subtract/1 -> Abs/1
  Constant/1 -> Subtract/2
  Weighted Sample Time/1 -> Subtract/1
  In/1 -> Weighted Sample Time/1

== system TxRxRFModel/ad9361_tx1/Analog_Filters_TX ==
  In : Inport
  " AnalogFilter " : dsparch4/Analog Filter Design  method=Butterworth  filttype=Lowpass  N=3  Wlo=1.6*ad9361_tx_pars.Fpass*2*pi  Whi=80  Rp=2  Rs=40
  AnalogFilter : dsparch4/Analog Filter Design  method=Butterworth  filttype=Lowpass  N=3  Wlo=1.6*ad9361_tx_pars.Fpass*2*pi  Whi=80  Rp=2  Rs=40
  "AnalogFilter " : dsparch4/Analog Filter Design  method=Butterworth  filttype=Lowpass  N=1  Wlo=5*ad9361_tx_pars.Fpass*2*pi  Whi=80  Rp=2  Rs=40
  AnalogFilters : dsparch4/Analog Filter Design  method=Butterworth  filttype=Lowpass  N=1  Wlo=5*ad9361_tx_pars.Fpass*2*pi  Whi=80  Rp=2  Rs=40
  Complex to Real-Imag : ComplexToRealImag
  Real : Outport
  Imaginary : Outport  Port=2
  wires:
  "AnalogFilter "/1 -> Real/1
  " AnalogFilter "/1 -> AnalogFilters/1
  AnalogFilter/1 -> "AnalogFilter "/1
  Complex to Real-Imag/2 -> " AnalogFilter "/1
  In/1 -> Complex to Real-Imag/1
  Complex to Real-Imag/1 -> AnalogFilter/1
  AnalogFilters/1 -> Imaginary/1

== system TxRxRFModel/ad9361_tx1/DUC_Filters_TX ==
  In : Inport
  Add : Sum
  Band-Limited White Noise : simulink/Sources/Band-Limited White Noise  Cov=[0.1]  Ts=ad9361_tx_pars.Tduc  seed=[23341]
  Hm1 : dspmlti4/FIR Interpolation  FilterSource=Filter object  h=designMultirateFIR(3,1)  L=3  FilterObject=ad9361_tx_pars.Hm1_tx  framing=Enforce single-rate processing  outputBufInitCond=0  roundingMode=Floor  overflowMode=off  firstCoeffDataTypeStr=Inherit: Same word length as input  firstCoeffMin=[]  firstCoeffMax=[]  firstCoeffLastDataTypeStr=Inherit: Same word length as input  outputDataTypeStr=Inherit: Same as accumulator  outputMin=[]  outputMax=[]  outputLastDataTypeStr=Inherit: Same as accumulator
      settings: SourceProductName=DSP System Toolbox
  Hm2 : dspmlti4/FIR Interpolation  FilterSource=Filter object  h=designMultirateFIR(3,1)  L=3  FilterObject=ad9361_tx_pars.Hm2_tx  framing=Enforce single-rate processing  outputBufInitCond=0  roundingMode=Floor  overflowMode=off  firstCoeffDataTypeStr=Inherit: Same word length as input  firstCoeffMin=[]  firstCoeffMax=[]  firstCoeffLastDataTypeStr=Inherit: Same word length as input  outputDataTypeStr=Inherit: Same as accumulator  outputMin=[]  outputMax=[]  outputLastDataTypeStr=Inherit: Same as accumulator
      settings: SourceProductName=DSP System Toolbox
  Hm3 : dspmlti4/FIR Interpolation  FilterSource=Filter object  h=designMultirateFIR(3,1)  L=3  FilterObject=ad9361_tx_pars.Hm3_tx  framing=Enforce single-rate processing  outputBufInitCond=0  roundingMode=Floor  overflowMode=off  firstCoeffDataTypeStr=Inherit: Same word length as input  firstCoeffMin=[]  firstCoeffMax=[]  firstCoeffLastDataTypeStr=Inherit: Same word length as input  outputDataTypeStr=Inherit: Same as accumulator  outputMin=[]  outputMax=[]  outputLastDataTypeStr=Inherit: Same as accumulator
      settings: SourceProductName=DSP System Toolbox
  Hmd : dspmlti4/FIR Interpolation  FilterSource=Filter object  h=fir1(15,1/4)  L=3  FilterObject=ad9361_tx_pars.Hmd_tx  framing=Allow multirate processing  outputBufInitCond=0  roundingMode=Floor  overflowMode=off  firstCoeffDataTypeStr=Inherit: Same word length as input  firstCoeffMin=[]  firstCoeffMax=[]  firstCoeffLastDataTypeStr=Inherit: Same word length as input  outputDataTypeStr=Inherit: Same as accumulator  outputMin=[]  outputMax=[]  outputLastDataTypeStr=Inherit: Same as accumulator
      settings: SourceProductName=DSP System Toolbox
  NoiseFloor : dspmathops/dB Gain  dB=-130-20-8  intype=Amplitude
      settings: SourceProductName=DSP System Toolbox  SourceProductBaseCode=DS
  Short : ad9361_private/Short  SystemSampleTime=-1  VariantControl=ad9361_tx_hm1Filt==0
  dB Gain : dspmathops/dB Gain  dB=log2(ad9361_tx_pars.BW_duc/ad9361_tx_pars.SamplingRate)*6  intype=Amplitude
      settings: SourceProductName=DSP System Toolbox  SourceProductBaseCode=DS
  Out : Outport
  wires:
  Hmd/1 -> Hm1/1
  Hm1/1 -> Hm2/1
  Hm3/1 -> Short/1
  In/1 -> Hmd/1
  dB Gain/1 -> Add/2
  Add/1 -> Out/1
  Band-Limited White Noise/1 -> NoiseFloor/1
  NoiseFloor/1 -> Add/1
  Short/1 -> dB Gain/1
  Hm2/1 -> Hm3/1

== system TxRxRFModel/ad9361_tx1/RF_TX ==
  note: NF, OIP3, S22
  note: Carrier Leakage
      | Gain Imbalance (SSB image)
  In_I : Inport
  In_Q : Inport  Port=2
  Attenuation : Inport  Port=3
  Amplifier_I : simrfV2elements/VGA  classname=vga  Zin=50  Zout=50  IO=Output  InternalGrounding=on
      settings: SourceProductName=RF Blockset  SourceProductBaseCode=RB
  Amplifier_I1 : simrfV2elements/VGA  classname=vga  Zin=50  Zout=50  IO=Output  InternalGrounding=on
      settings: SourceProductName=RF Blockset  SourceProductBaseCode=RB
  Configuration : simrfV2util1/Configuration  AutoFreq=off  Tones=RF Hz  Harmonics=3  NormalizeCarrierPower=on  SolverType=Auto  UseCCode=on  StepSize=Tstep s  AddNoise=on  defaultRNG=on  Seed=0  Temperature=290.0 K  SolverDelFlag=0  AbsTol=1e-6  RelTol=1e-3  MaxIter=10  ErrorEstimationType=2-norm over all variables
      settings: SourceProductName=RF Blockset  SourceProductBaseCode=RB
  Constant2 : Constant  Value=inf
  Display : Display
      settings: Decimation=100
  Gain1 : Gain  Gain=-1
  Inport_I : simrfV2util1/Inport  SimulinkInputSignalType=Power  CarrierFreq=0 Hz  ZS=50  InternalGrounding=on
      settings: SourceProductName=RF Blockset  SourceProductBaseCode=RB
  Inport_Q : simrfV2util1/Inport  SimulinkInputSignalType=Power  CarrierFreq=0 Hz  ZS=50  InternalGrounding=on
      settings: SourceProductName=RF Blockset  SourceProductBaseCode=RB
  Modulator : Subsystem
  Outport : simrfV2util1/Outport  SensorType=Power  OutputFormat=Complex Baseband  CarrierFreq=RF Hz  ZL=50  InternalGrounding=on  StepSize=-1 s  AutoStep=off
      settings: SourceProductName=RF Blockset  SourceProductBaseCode=RB
  PA : Subsystem
  Quantizer : Quantizer  QuantizationInterval=0.25
  Saturation : Saturate  UpperLimit=89.75  LowerLimit=0
  Out : Outport
  wires:
  In_I/1 -> Inport_I/1
  In_Q/1 -> Inport_Q/1
  Attenuation/1 -> Quantizer/1
  Saturation/1 -> PA/1(" Attenuation"), Display/1, Modulator/1(Attenuation), Gain1/1
  Quantizer/1 -> Saturation/1
  Outport/1 -> Out/1
  Constant2/1 -> Amplifier_I1/3, Amplifier_I1/2, Amplifier_I/3, Amplifier_I/2
  Gain1/1 -> Amplifier_I1/1, Amplifier_I/1
  connections:
  Amplifier_I/LConn1 -- Inport_I/RConn1
  Inport_Q/RConn1 -- Amplifier_I1/LConn1
  Amplifier_I1/RConn1 -- Modulator/LConn2
  Outport/LConn1 -- Configuration/LConn1 -- PA/RConn1
  PA/LConn1 -- Modulator/RConn1
  Modulator/LConn1 -- Amplifier_I/RConn1

== system TxRxRFModel/ad9361_tx1/VerifySampleTime ==
  In : Inport
  Abs : Abs
  Assertion : Assertion  AssertionFailFcn=errordlg('Test signal sample time and I/Q sample rate are not consistent');
  Compare To Constant : simulink/Logic and Bit Operations/Compare To Constant  relop=<=  const=eps(1/ad9361_tx_pars.SamplingRate)*1e12  OutDataTypeStr=boolean
  Constant : Constant  Value=1/ad9361_tx_pars.SamplingRate
  Subtract : Sum  Inputs=+-
  Weighted Sample Time : SampleTimeMath  TsampMathOp=Ts Only
  wires:
  Abs/1 -> Compare To Constant/1
  In/1 -> Weighted Sample Time/1
  Weighted Sample Time/1 -> Subtract/1
  Constant/1 -> Subtract/2
  Subtract/1 -> Abs/1
  Compare To Constant/1 -> Assertion/1

== system TxRxRFModel/Receiver/CRC Check and DMA Pack/CRC Check ES ==
  note: NOTE:
      | 	The Valid signal must be latched during a packet, which is
      | 	a bug.  Therefore we must use the CRC block in an enabled
      | 	subsystem
  note: CRC Requires
      | Always High
      | Valid Signal During
      | Packet
  Valid : Inport
  Bits : Inport  Port=2
  endCRC : Inport  Port=3
  StartData : Inport  Port=4
  payloadLen : Inport  Port=5
  Enable : EnablePort
  CRC Decode Lag : Delay  DelayLength=crcDecodeLag
  Check CRC Result (DEBUG) : MATLAB Function  Commented=on  TreatAsAtomicUnit=on
  Convert To fi : DataTypeConversion  OutDataTypeStr=fixdt(0,1,0)  SaturateOnIntegerOverflow=on
  Debug CRC input : MATLAB Function  Commented=on  TreatAsAtomicUnit=on
  General CRC Syndrom Detector HDL Optimized : commcrc2/General CRC Syndrome Detector HDL Optimized  Polynomial=crc32Poly  InitialState=0  DirectMethod=off  ReflectInput=off  ReflectCRCChecksum=off  FinalXORValue=0  SimulateUsing=Code generation
      settings: SourceProductName=Communications System Toolbox  SourceProductBaseCode=CM
  dataOut : Outport  InitialOutput=0
  startOut : Outport  Port=2  InitialOutput=0
  endOut : Outport  Port=3  InitialOutput=0
  validOut : Outport  Port=4  InitialOutput=0
  err : Outport  Port=5  InitialOutput=0
  payloadLenOut : Outport  Port=6  InitialOutput=0
  wires:
  Bits/1 -> Convert To fi/1, Debug CRC input/1(u)
  General CRC Syndrom Detector HDL Optimized/1 -> Check CRC Result (DEBUG)/1(bits), dataOut/1
  General CRC Syndrom Detector HDL Optimized/3 -> Check CRC Result (DEBUG)/3(done), endOut/1
  General CRC Syndrom Detector HDL Optimized/4 -> Check CRC Result (DEBUG)/4(valid), validOut/1
  General CRC Syndrom Detector HDL Optimized/5 -> Check CRC Result (DEBUG)/5(err), err/1
  General CRC Syndrom Detector HDL Optimized/2 -> Check CRC Result (DEBUG)/2(start), startOut/1
  Convert To fi/1 -> General CRC Syndrom Detector HDL Optimized/1
  payloadLen/1 -> CRC Decode Lag/1
  CRC Decode Lag/1 -> payloadLenOut/1
  StartData/1 -> Debug CRC input/4(startFlag), General CRC Syndrom Detector HDL Optimized/2
  endCRC/1 -> Debug CRC input/3(endFlag), General CRC Syndrom Detector HDL Optimized/3
  Valid/1 -> General CRC Syndrom Detector HDL Optimized/4, Debug CRC input/2(enable)

== system TxRxRFModel/Receiver/CRC Check and DMA Pack/DMA Interface ==
  bitIn : Inport
  startIn : Inport  Port=2
  endIn : Inport  Port=3
  validIn : Inport  Port=4
  err : Inport  Port=5
  payloadLen : Inport  Port=6
  Bit Packer : MATLAB Function  TreatAsAtomicUnit=on
  Convert Payload Length To Bytes : Subsystem
  Data Type Conversion : DataTypeConversion  OutDataTypeStr=boolean
  Delay : Delay  DelayLength=1
  Delay Error To Last Byte of Out : Delay  DelayLength=1
  Display : Display
  byteOut : Outport
  validOut : Outport  Port=2
  sync : Outport  Port=3
  payloadLenOut : Outport  Port=4
  wires:
  bitIn/1 -> Data Type Conversion/1
  Delay/1 -> Bit Packer/3(endIn)
  Delay Error To Last Byte of Out/1 -> Bit Packer/4(err)
  Bit Packer/2(validOut) -> validOut/1
  Bit Packer/3(startOut) -> sync/1
  Bit Packer/1(byteOut) -> Display/1, byteOut/1
  err/1 -> Delay Error To Last Byte of Out/1
  validIn/1 -> Bit Packer/5(validIn)
  endIn/1 -> Delay/1
  startIn/1 -> Bit Packer/2(startIn)
  Data Type Conversion/1 -> Bit Packer/1(bitIn)
  payloadLen/1 -> Convert Payload Length To Bytes/1(In1)
  Convert Payload Length To Bytes/1(Out1) -> payloadLenOut/1
